simulink model "lab_7b"  (R2016a)
settings: Solver=VariableStepAuto  StartTime=0.0  StopTime=10.0  RelTol=1e-3
undefined symbols (not defined in the file): DiscIntNeverNeededParam
libraries: dsparch4 x1, commsynccomp2 x1, dspsrcs4 x1
settings Model: Creator=Sahilur Rahman  LastModifiedBy=Sahilur Rahman

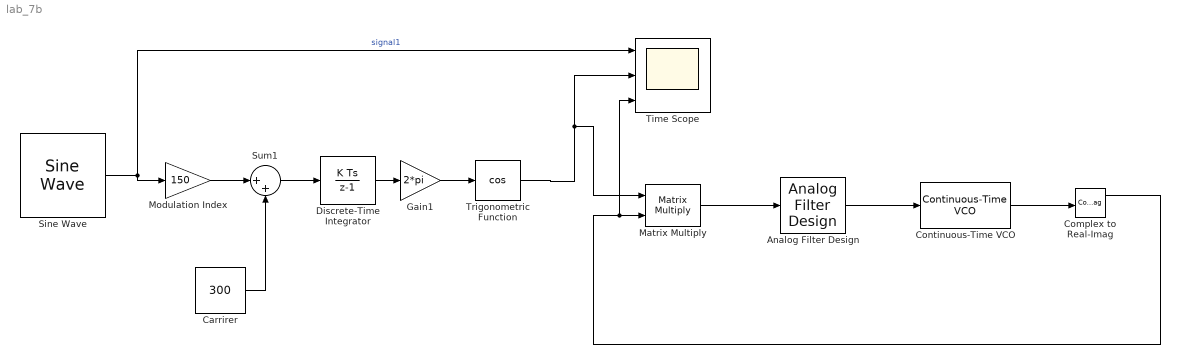
== system lab_7b ==
  Analog Filter Design : dsparch4/Analog Filter Design  method=Butterworth  filttype=Lowpass  N=10  Wlo=2*pi*10  Whi=80  Rp=2  Rs=40
  Carrirer : Constant  Value=300
  Complex to Real-Imag : ComplexToRealImag
  Continuous-Time VCO : commsynccomp2/Continuous-Time VCO  Ac=1  Fc=10  Kc=50  Ph=0
  Discrete-Time Integrator : DiscreteIntegrator  gainval=1  InitialConditionSetting=State (most efficient)  SampleTime=1/98000  ICPrevOutput=DiscIntNeverNeededParam  ICPrevScaledInput=DiscIntNeverNeededParam
  Gain1 : Gain  Gain=2*pi
  Matrix Multiply : Product  Multiplication=Matrix(*)
  Modulation Index : Gain  Gain=150
  Sine Wave : dspsrcs4/Sine Wave  Amplitude=1  Frequency=10  Phase=90  SampleMode=Discrete  OutComplex=Real  CompMethod=Trigonometric fcn  TableSize=Speed  SampleTime=1/98000  SamplesPerFrame=1  ResetState=Restart at time zero  OutputFrames=off  dataType=double  wordLen=16  udDataType=sfix(16)  fracBitsMode=Best precision  numFracBits=15  OutDataTypeStr=double  LastOutDataTypeStr=double
  Sum1 : Sum  Inputs=|++
  Time Scope : Scope  NumInputPorts=3
  Trigonometric Function : Trigonometry  Operator=cos
  wires:
  Sine Wave/1 -> Modulation Index/1, Time Scope/1  "signal1"
  Modulation Index/1 -> Sum1/1
  Sum1/1 -> Discrete-Time Integrator/1
  Discrete-Time Integrator/1 -> Gain1/1
  Gain1/1 -> Trigonometric Function/1
  Carrirer/1 -> Sum1/2
  Analog Filter Design/1 -> Continuous-Time VCO/1
  Continuous-Time VCO/1 -> Complex to Real-Imag/1
  Matrix Multiply/1 -> Analog Filter Design/1
  Complex to Real-Imag/1 -> Time Scope/3, Matrix Multiply/2
  Trigonometric Function/1 -> Matrix Multiply/1, Time Scope/2
